simulink model "nonlin_quad_plant"  (R2024a)
settings: Solver=VariableStepAuto  StartTime=0.0  StopTime=10  FixedStep=sample_time  RelTol=1e-3
values from neighbouring files (symbols this model uses):
  drag_mat = [kdx 0 0; 0 kdy 0; 0 0 kdz]    [non_lin_plant.m]
  g = 9.81    [non_lin_plant.m]
  J = [inertia_xx; inertia_yy; inertia_zz]    [non_lin_plant.m]
  Jr = 0.044    [non_lin_plant.m]
  Kd = 1.3858e-6    (= 1.3858e-06)    [non_lin_plant.m]
  Kt = 1.3328e-5    (= 1.3328e-05)    [non_lin_plant.m]
  L = 0.56    [non_lin_plant.m]
  m = 1.4    [non_lin_plant.m]
  max_mot_speed = 925    [non_lin_plant.m]
settings Model: Creator=Lorenzo-Desk  LastModifiedBy=loca

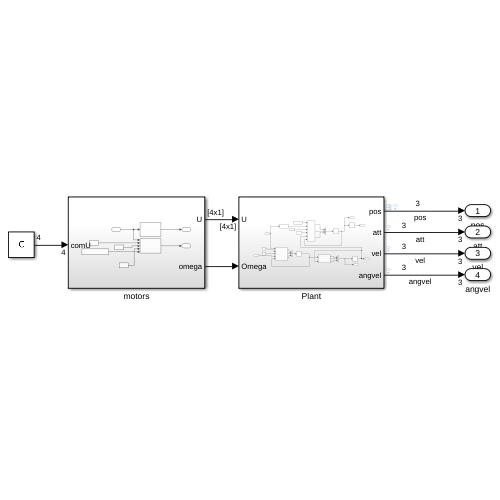
[thumbnail: Simulink's stored preview of the top-level diagram]
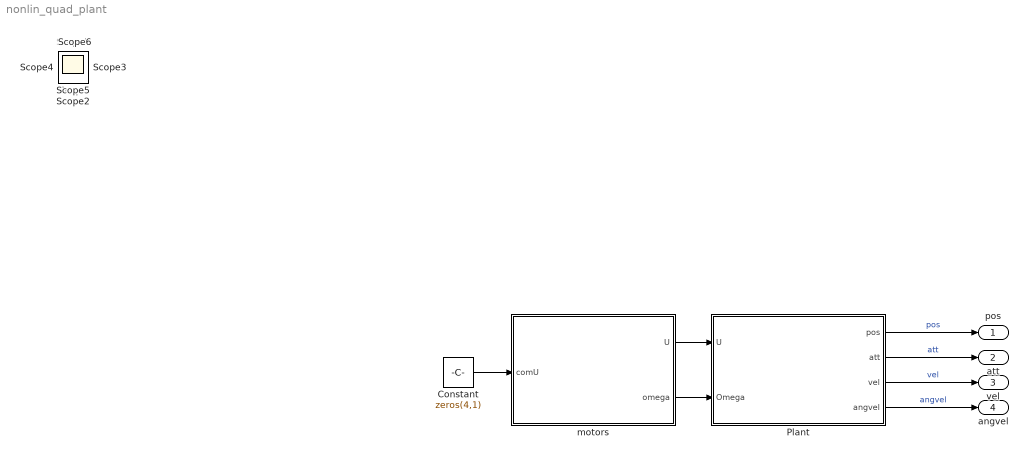
== system nonlin_quad_plant ==
  Constant : Constant  Value=zeros(4,1)
  Plant : Subsystem
  motors : Subsystem
  pos : Outport
  att : Outport  Port=2
  vel : Outport  Port=3
  angvel : Outport  Port=4
  Scope{,1..6} (7 alike) : Scope
  wires:
  Plant/1(pos) -> pos/1  "pos"
  Plant/2(att) -> att/1  "att"
  Plant/3(vel) -> vel/1  "vel"
  Plant/4(angvel) -> angvel/1  "angvel"
  motors/1(U) -> Plant/1(U)
  motors/2(omega) -> Plant/2(Omega)
  Constant/1 -> motors/1(comU)

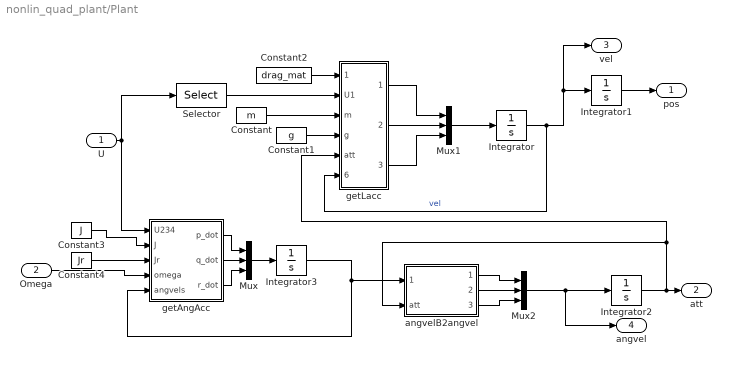
== system nonlin_quad_plant/Plant ==
  U : Inport
  Omega : Inport  Port=2
  Constant : Constant  Value=m
  Constant1 : Constant  Value=g
  Constant2 : Constant  Value=drag_mat
  Constant3 : Constant  Value=J
  Constant4 : Constant  Value=Jr
  Integrator{,1..3} (4 alike) : Integrator
  Mux : Mux  Inputs=3
  Mux1 : Mux  Inputs=3
  Mux2 : Mux  Inputs=3
  Selector : Selector  InputPortWidth=4  IndexOptions=Index vector (dialog)  Indices=[1]  OutputSizes=1
  angvelB2angvel : MATLAB Function  TreatAsAtomicUnit=on
  getAngAcc : MATLAB Function  TreatAsAtomicUnit=on
  getLacc : MATLAB Function  TreatAsAtomicUnit=on
  pos : Outport
  att : Outport  Port=2
  vel : Outport  Port=3
  angvel : Outport  Port=4
  wires:
  Integrator/1 -> getLacc/6(vels), vel/1, Integrator1/1  "vel"
  Integrator1/1 -> pos/1
  Integrator2/1 -> getLacc/5(att), angvelB2angvel/2(att), att/1
  Integrator3/1 -> getAngAcc/5(angvels), angvelB2angvel/1(angvelB)
  Selector/1 -> getLacc/2(U1)
  U/1 -> getAngAcc/1(U234), Selector/1
  Omega/1 -> getAngAcc/4(omega)
  Constant/1 -> getLacc/3(m)
  Constant1/1 -> getLacc/4(g)
  Constant2/1 -> getLacc/1(drag_mat)
  Constant3/1 -> getAngAcc/2(J)
  Mux/1 -> Integrator3/1
  getAngAcc/2(q_dot) -> Mux/2
  getAngAcc/1(p_dot) -> Mux/1
  getAngAcc/3(r_dot) -> Mux/3
  Constant4/1 -> getAngAcc/3(Jr)
  Mux1/1 -> Integrator/1
  getLacc/2(y_ddot) -> Mux1/2
  getLacc/1(x_ddot) -> Mux1/1
  getLacc/3(z_ddot) -> Mux1/3
  Mux2/1 -> angvel/1, Integrator2/1
  angvelB2angvel/1(phi_dot) -> Mux2/1
  angvelB2angvel/2(theta_dot) -> Mux2/2
  angvelB2angvel/3(psi_dot) -> Mux2/3

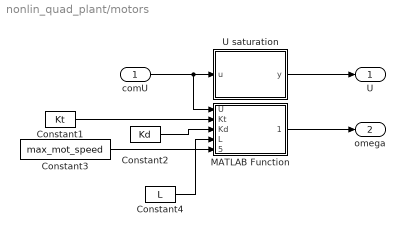
== system nonlin_quad_plant/motors ==
  comU : Inport
  Constant1 : Constant  Value=Kt
  Constant2 : Constant  Value=Kd
  Constant3 : Constant  Value=max_mot_speed
  Constant4 : Constant  Value=L
  MATLAB Function : MATLAB Function  TreatAsAtomicUnit=on
  U saturation : MATLAB Function  TreatAsAtomicUnit=on
  U : Outport
  omega : Outport  Port=2
  wires:
  Constant3/1 -> MATLAB Function/5(max_mot_speed)
  Constant2/1 -> MATLAB Function/3(Kd)
  MATLAB Function/1(omega) -> omega/1
  Constant1/1 -> MATLAB Function/2(Kt)
  comU/1 -> U saturation/1(u), MATLAB Function/1(U)
  U saturation/1(y) -> U/1
  Constant4/1 -> MATLAB Function/4(L)

== matlab function nonlin_quad_plant/motors/U saturation ==
  data: u input; y output
function y = fcn(u)

y = u;

== matlab function nonlin_quad_plant/motors/MATLAB Function ==
  data: U input; omega output; Kt input; Kd input; L input; max_mot_speed input
function omega = fcn(U, Kt, Kd, L , max_mot_speed)
U1 = U(1); U2 = U(2); U3 = U(3); U4 = U(4);
%% Get motor speeds
W = zeros(4,1);
W(1) = sqrt(U1/(4*Kt) + U3/(2*Kt*L) + U4/(4*Kd));
W(2) = sqrt(U1/(4*Kt) - U2/(2*Kt*L) - U4/(4*Kd));
W(3) = sqrt(U1/(4*Kt) - U3/(2*Kt*L) + U4/(4*Kd));
W(4) = sqrt(U1/(4*Kt) + U2/(2*Kt*L) - U4/(4*Kd));

for i = 1:4
    if W(i)>max_mot_speed
        W(i) = max_mot_speed;
    end
end

omega = W(1) - W(2) + W(3) - W(4);

== matlab function nonlin_quad_plant/Plant/getLacc ==
  data: drag_mat input; U1 input; m input; g input; att input; vels input; x_ddot output; y_ddot output; z_ddot output
function [x_ddot, y_ddot, z_ddot] = fcn(drag_mat, U1, m, g, att, vels)
phi = att(1); theta = att(2); psi = att(3);
Kdx = drag_mat(1,1); Kdy = drag_mat(2,2); Kdz = drag_mat(3,3);
x_dot = vels(1); y_dot = vels(2); z_dot = vels(3);
% Linear Acceleratios
x_ddot = 1/m * (-U1*(cos(phi)*sin(theta)*cos(psi)+sin(phi)*sin(psi))-Kdx*x_dot);
y_ddot = 1/m * (-U1*(cos(phi)*sin(theta)*sin(psi)-cos(psi)*sin(phi))-Kdy*y_dot);
z_ddot = -1/m*(U1*cos(phi)*cos(theta)-Kdz*z_dot)+g;

== matlab function nonlin_quad_plant/Plant/getAngAcc ==
  data: U234 input; J input; Jr input; p_dot output; omega input; angvels input; q_dot output; r_dot output
function [p_dot, q_dot, r_dot] = fcn(U234, J, Jr, omega, angvels)
Jx = J(1); Jy = J(2); Jz = J(3);
U2 = U234(2); U3 = U234(3); U4 = U234(4);
p = angvels(1); q = angvels(2); r = angvels(3);
% Angle Accelerations
p_dot = 1/Jx * (q*r*(Jy-Jz) - Jr*q*omega + U2);
q_dot = 1/Jy * (p*r*(Jz-Jx) - Jr*p*omega + U3);
r_dot = 1/Jz * (p*q*(Jx-Jy) + U4);

== matlab function nonlin_quad_plant/Plant/angvelB2angvel ==
  data: angvelB input; phi_dot output; att input; theta_dot output; psi_dot output
function [phi_dot, theta_dot, psi_dot] = fcn(angvelB, att)
p = angvelB(1); q = angvelB(2); r = angvelB(3);
phi = att(1); theta = att(2); psi = att(3);
% Angle Rates
phi_dot = p + q*sin(phi)*tan(theta) + r*cos(phi)*tan(theta);
theta_dot = q*cos(phi) - r*sin(phi);
psi_dot = q*sin(phi)/cos(theta) + r*cos(phi)/cos(theta);
